simulink model "cp_model"  (Simulink 8.6)
settings: Solver=ode45  StartTime=-50  StopTime=300  FixedStep=.01  RelTol=1e-3
undefined symbols (not defined in the file or in its folder): paux
settings Model: Creator=Roberto  LastModifiedBy=eleonora.grespan
settings DataIOCC: LimitDataPoints=off  SaveOutput=off  SignalLogging=off  DSMLogging=off  SaveTime=off  ReturnWorkspaceOutputsName=simOut
settings DebuggingCC: SolverPrmCheckMsg=none  FcnCallInpInsideContextMsg=UseLocalSettings

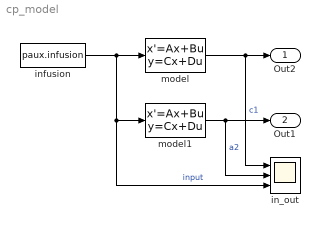
== system cp_model ==
  in_out : Scope  NumInputPorts=3
  infusion : FromWorkspace  VariableName=paux.infusion  SampleTime=0  OutputAfterFinalValue=Holding final value
  model : StateSpace  A="[-paux.a 0; 0  -paux.b]"  B=[1;1]  C=[paux.A paux.B];  D=0  X0=[paux.ISRb/paux.a; paux.ISRb/paux.b]  ContinuousStateAttributes='output'
  model1 : StateSpace  A="[-paux.a 0; 0  -paux.b]"  B=[1;1]  C=[paux.A paux.B]  D=0  X0=[paux.ISRb/paux.a; paux.ISRb/paux.b]  ContinuousStateAttributes='output'
  Out2 : Outport
  Out1 : Outport  Port=2
  wires:
  model/1 -> Out2/1, in_out/1  "c1"
  infusion/1 -> in_out/3, model1/1, model/1  "input"
  model1/1 -> Out1/1, in_out/2  "a2"
